simulink model "HW6a"  (R2020b)
settings: Solver=ode23  StartTime=0.0  StopTime=50  FixedStep=0.05  RelTol=1e-3  AbsTol=1e-6  EnableMultiTasking=on
InitFcn:
  | gamma1 = 1
  | gamma2 = 1
settings Model: ExtModeTrigMode=oneshot  ExtModeArmWhenConnect=off  ExtModeAutoUpdateStatusClock=off  Creator=mstefano  LastModifiedBy=jrsco
settings SolverCC: AutoScaleAbsTol=off
settings DataIOCC: SaveFormat=Array  ReturnWorkspaceOutputs=off
settings OptimizationCC: BlockReduction=off  BooleanDataType=off  ExpressionDepthLimit=2147483647  InitFltsAndDblsToZero=on  LifeSpan=inf
settings DebuggingCC: SaveWithParameterizedLinksMsg=none  UnderspecifiedInitializationDetection=Classic  MergeDetectMultiDrivingBlocksExec=none  SignalResolutionControl=TryResolveAllWithWarning  MultiTaskDSMMsg=warning  MultiTaskCondExecSysMsg=none  FcnCallInpInsideContextMsg=warning  StateNameClashWarn=warning  SFUnexpectedBacktrackingDiag=warning  SFNoUnconditionalDefaultTransitionDiag=warning  SFExecutionAtInitializationDiag=none  ArithmeticOperatorsInVariantConditions=warning
settings HardwareCC: ProdBitPerPointer=32  ProdBitPerSizeT=32  ProdBitPerPtrDiffT=32  ProdLargestAtomicFloat=None  ProdIntDivRoundTo=Undefined  ProdEndianess=Unspecified  ProdWordSize=32  ProdHWDeviceType=32-bit Generic  TargetUnknown=on
settings ModelReferenceCC: PropagateSignalLabelsOutOfModel=off
settings SFSimCC: SimUseLocalCustomCode=off  CustomCodeUndefinedFunction=UseInterfaceOnly
settings RTWCC: RTWUseLocalCustomCode=off
settings CodeAppCC: StateflowObjectComments=on
settings GRTTargetCC: TargetFcnLib=ansi_tfl_tmw.mat  TargetLangStandard=C89/C90 (ANSI)  ModelReferenceCompliant=off  CompOptLevelCompliant=off  CombineOutputUpdateFcns=off  MatFileLogging=off  GRTInterface=on
settings ConfigComp: CovMetricSettings=dw  CovSaveCumulativeToWorkspaceVar=on  CovSaveSingleToWorkspaceVar=on  CovExternalEMLEnable=off

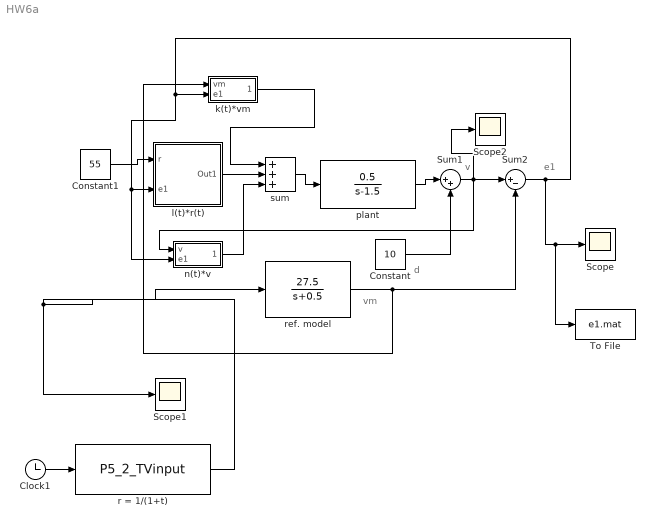
== system HW6a ==
  note: vm
  note: v
  note: e1
  note: d
  Clock1 : Clock
  Constant : Constant  Value=10
  Constant1 : Constant  Value=55
  Scope : Scope
  Scope1 : Scope
  Scope2 : Scope
  Sum1 : Sum  Inputs=|++  InputSameDT=on  SaturateOnIntegerOverflow=on  OutDataTypeStr=Inherit: Same as first input
  Sum2 : Sum  Inputs=|+-  InputSameDT=on  SaturateOnIntegerOverflow=on  OutDataTypeStr=Inherit: Same as first input
  To File : ToFile  Filename=e1.mat  MatrixName=e1
  k(t)*vm : Subsystem
  l(t)*r(t) : Subsystem
  n(t)*v : Subsystem
  plant : TransferFcn  Numerator=[0.5]  Denominator=[1 -1.5]
  r = 1/(1+t) : S-Function  FunctionName=P5_2_TVinput  SFunctionDeploymentMode=off  EnableBusSupport=off
  ref. model : TransferFcn  Numerator=[27.5]  Denominator=[1 0.5]
  sum : Sum  Inputs=+++  InputSameDT=on  SaturateOnIntegerOverflow=on  OutDataTypeStr=Inherit: Same as first input
  wires:
  sum/1 -> plant/1
  k(t)*vm/1(Out1) -> sum/1
  l(t)*r(t)/1(Out1) -> sum/2
  ref. model/1 -> k(t)*vm/1(vm), Sum2/2
  Sum2/1 -> n(t)*v/2(e1), l(t)*r(t)/2(e1), k(t)*vm/2(e1), Scope/1, To File/1
  Clock1/1 -> r = 1/(1+t)/1
  r = 1/(1+t)/1 -> Scope1/1, ref. model/1
  Constant/1 -> Sum1/2
  plant/1 -> Sum1/1
  Sum1/1 -> Scope2/1, n(t)*v/1(v), Sum2/1
  Constant1/1 -> l(t)*r(t)/1(r)
  n(t)*v/1(Out1) -> sum/3

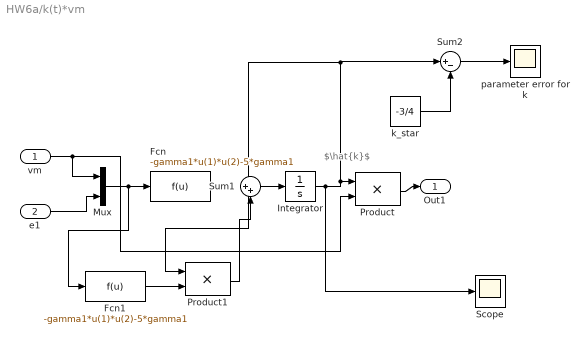
== system HW6a/k(t)*vm ==
  note: $\hat{k}$
  vm : Inport
  e1 : Inport  Port=2
  Fcn : Fcn  Expr=-gamma1*u(1)*u(2)-5*gamma1
  Fcn1 : Fcn  Expr=-gamma1*u(1)*u(2)-5*gamma1
  Integrator : Integrator  InitialCondition=0.1
  Mux : Mux  Inputs=2
  Product : Product  InputSameDT=on  RndMeth=Zero  SaturateOnIntegerOverflow=on  OutDataTypeStr=Inherit: Same as first input
  Product1 : Product  InputSameDT=on  RndMeth=Zero  SaturateOnIntegerOverflow=on  OutDataTypeStr=Inherit: Same as first input
  Scope : Scope
  Sum1 : Sum  Inputs=|++  InputSameDT=on  SaturateOnIntegerOverflow=on  OutDataTypeStr=Inherit: Same as first input
  Sum2 : Sum  Inputs=|+-  InputSameDT=on  SaturateOnIntegerOverflow=on  OutDataTypeStr=Inherit: Same as first input
  k_star : Constant  Value=-3/4
  parameter error for k : Scope
  Out1 : Outport
  wires:
  vm/1 -> Product/2, Mux/1
  e1/1 -> Mux/2
  Mux/1 -> Fcn1/1, Fcn/1
  Product/1 -> Out1/1
  Integrator/1 -> Scope/1, Product1/1, Sum2/1, Product/1
  Sum2/1 -> parameter error for k/1
  k_star/1 -> Sum2/2
  Fcn1/1 -> Product1/2
  Sum1/1 -> Integrator/1
  Product1/1 -> Sum1/2

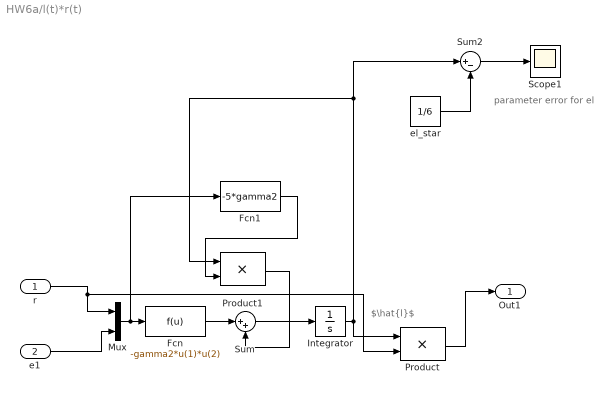
== system HW6a/l(t)*r(t) ==
  note: $\hat{l}$
  note: parameter error for el
  r : Inport
  e1 : Inport  Port=2
  Fcn : Fcn  Expr=-gamma2*u(1)*u(2)
  Fcn1 : Fcn  Expr=-5*gamma2
  Integrator : Integrator  InitialCondition=0.1
  Mux : Mux  Inputs=2
  Product : Product  InputSameDT=on  RndMeth=Zero  SaturateOnIntegerOverflow=on  OutDataTypeStr=Inherit: Same as first input
  Product1 : Product  InputSameDT=on  RndMeth=Zero  SaturateOnIntegerOverflow=on  OutDataTypeStr=Inherit: Same as first input
  Scope1 : Scope
  Sum : Sum  Inputs=|++
  Sum2 : Sum  Inputs=|+-  InputSameDT=on  SaturateOnIntegerOverflow=on  OutDataTypeStr=Inherit: Same as first input
  el_star : Constant  Value=1/6
  Out1 : Outport
  wires:
  r/1 -> Mux/1, Product/2
  e1/1 -> Mux/2
  Mux/1 -> Fcn1/1, Fcn/1
  Product/1 -> Out1/1
  Sum2/1 -> Scope1/1
  el_star/1 -> Sum2/2
  Integrator/1 -> Product1/1, Sum2/1, Product/1
  Fcn1/1 -> Product1/2
  Fcn/1 -> Sum/1
  Product1/1 -> Sum/2
  Sum/1 -> Integrator/1

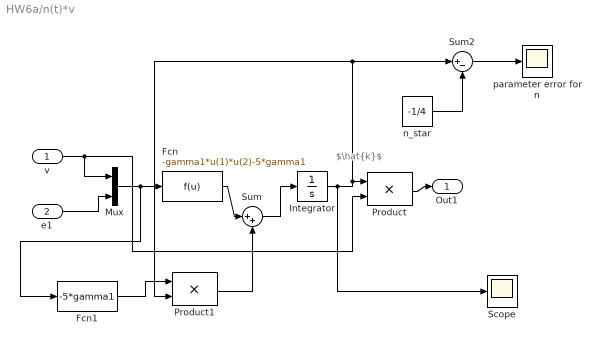
== system HW6a/n(t)*v ==
  note: $\hat{k}$
  v : Inport
  e1 : Inport  Port=2
  Fcn : Fcn  Expr=-gamma1*u(1)*u(2)-5*gamma1
  Fcn1 : Fcn  Expr=-5*gamma1
  Integrator : Integrator  InitialCondition=0.1
  Mux : Mux  Inputs=2
  Product : Product  InputSameDT=on  RndMeth=Zero  SaturateOnIntegerOverflow=on  OutDataTypeStr=Inherit: Same as first input
  Product1 : Product  InputSameDT=on  RndMeth=Zero  SaturateOnIntegerOverflow=on  OutDataTypeStr=Inherit: Same as first input
  Scope : Scope
  Sum : Sum  Inputs=|++
  Sum2 : Sum  Inputs=|+-  InputSameDT=on  SaturateOnIntegerOverflow=on  OutDataTypeStr=Inherit: Same as first input
  n_star : Constant  Value=-1/4
  parameter error for n : Scope
  Out1 : Outport
  wires:
  v/1 -> Product/2, Mux/1
  e1/1 -> Mux/2
  Mux/1 -> Fcn1/1, Fcn/1
  Product/1 -> Out1/1
  Integrator/1 -> Scope/1, Sum2/1, Product1/2, Product/1
  Sum2/1 -> parameter error for n/1
  n_star/1 -> Sum2/2
  Fcn1/1 -> Product1/1
  Fcn/1 -> Sum/1
  Product1/1 -> Sum/2
  Sum/1 -> Integrator/1
